simulink model "q_test_q2_usb"  (R2014b)
settings: Solver=FixedStepDiscrete  StartTime=0.0  StopTime=inf  FixedStep=0.002  RelTol=1e-3
PostLoadFcn:
  | qc_set_target_type(getConfigSet(bdroot, 'QUARC Default Target Configuration'));
undefined symbols (not defined in the file or in its folder): HIL, K_ENC, qc_get_step_size
libraries: quarc_library x12
settings Model: SimulationMode=external  ExtModeTrigDuration=5000  Creator=user  LastModifiedBy=amolki
settings SolverCC: PositivePriorityOrder=on
settings DataIOCC: SignalLoggingSaveFormat=ModelDataLogs
settings OptimizationCC: InitFltsAndDblsToZero=on
settings DebuggingCC: SaveWithParameterizedLinksMsg=none  UnderspecifiedInitializationDetection=Classic  MergeDetectMultiDrivingBlocksExec=none  MultiTaskDSMMsg=warning  MultiTaskCondExecSysMsg=none  FcnCallInpInsideContextMsg=UseLocalSettings  FrameProcessingCompatibilityMsg=error  StateNameClashWarn=warning
settings RTWCC: SystemTargetFile=quarc_win64.tlc  TemplateMakefile=quarc_default_tmf  Description=QUARC Win64 Target  ProcessScript=quarc_win64_make_rtw_hook
settings STFCustomTargetCC: TargetPreCompLibLocation=C:\PROGRA~3\QUARC\lib\2014b\win64\release  CodeReplacementLibrary=ANSI_C  ConcurrentExecutionCompliant=on  GeneratePreprocessorConditionals=Disable all  CombineOutputUpdateFcns=on  GRTInterface=off  SystemTargetFile=quarc_win64.tlc
settings GRTTargetCC: TargetPreCompLibLocation=C:\PROGRA~3\QUARC\lib\2014b\win64\release  CodeReplacementLibrary=ANSI_C  ParMdlRefBuildCompliant=off  CompOptLevelCompliant=off  MatFileLogging=off  CPPClassGenCompliant=off  ExtMode=on  ExtModeMexFile=quarc_comm

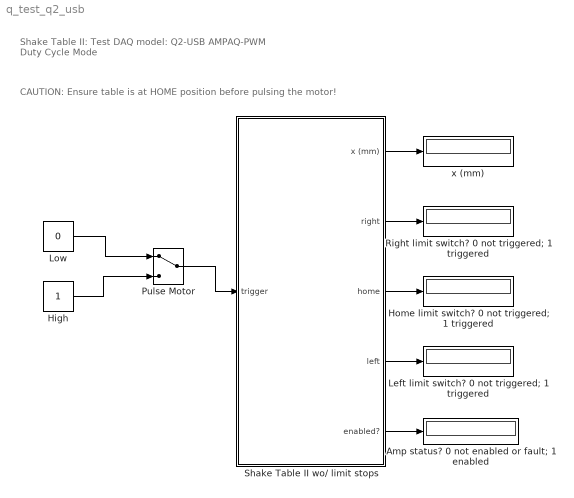
== system q_test_q2_usb ==
  note: Shake Table II: Test
      | DAQ model: Q2-USB
      | AMPAQ-PWM Duty Cycle Mode
  note: CAUTION: Ensure table is at HOME position before pulsing the motor!
  Amp status? 0 not enabled or fault; 1 enabled : Display
  High : Constant
  Home limit switch? 0 not triggered; 1 triggered : Display
  Left limit switch? 0 not triggered; 1 triggered : Display
  Low : Constant  Value=0
  Pulse Motor : ManualSwitch
  Right limit switch? 0 not triggered; 1 triggered : Display
  Shake Table II wo/ limit stops : Subsystem
  x (mm) : Display
  wires:
  Shake Table II wo/ limit stops/1(x (mm)) -> x (mm)/1
  Low/1 -> Pulse Motor/1
  High/1 -> Pulse Motor/2
  Shake Table II wo/ limit stops/2(right) -> Right limit switch? 0 not triggered; 1 triggered/1
  Shake Table II wo/ limit stops/4(left) -> Left limit switch? 0 not triggered; 1 triggered/1
  Shake Table II wo/ limit stops/3(home) -> Home limit switch? 0 not triggered; 1 triggered/1
  Shake Table II wo/ limit stops/5(enabled?) -> Amp status? 0 not enabled or fault; 1 enabled/1
  Pulse Motor/1 -> Shake Table II wo/ limit stops/1(trigger)

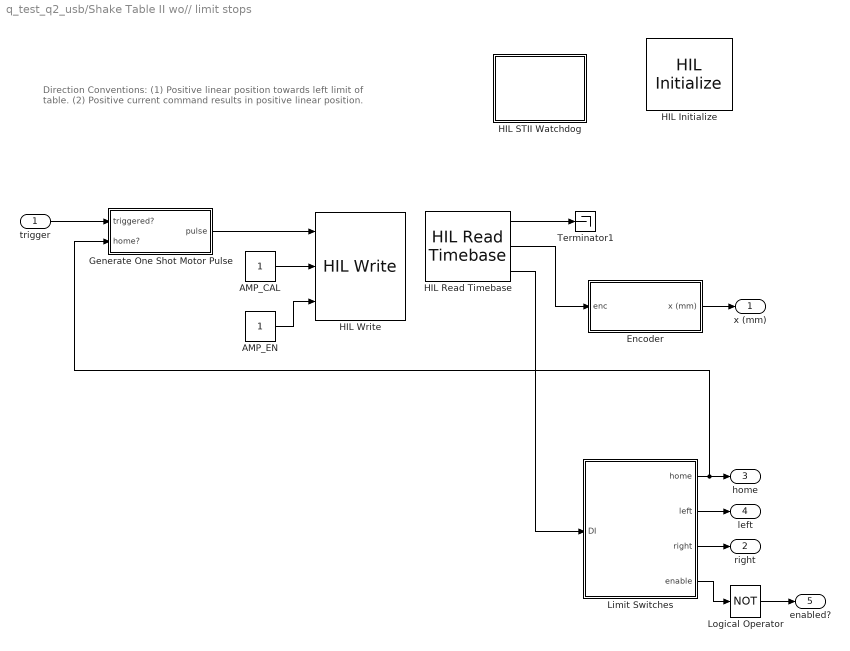
== system q_test_q2_usb/Shake Table II wo// limit stops ==
  note: Direction Conventions:
      | (1) Positive linear position towards left limit of table.
      | (2) Positive current command results in positive linear position.
  trigger : Inport
  AMP_CAL : Constant
  AMP_EN : Constant
  Encoder : Subsystem
  Generate One Shot Motor Pulse : Subsystem
  HIL Initialize : quarc_library/Data Acquisition/Generic/Configuration/HIL Initialize  object_name=HIL-1  board_type=q2_usb  board_number=0  board_options=d0=digital;d1=digital;led=auto;update_rate=fast;decimation=1  exclusive=off  active=on  hardware_clocks=[0]  clock_modes=[]  initial_clock_frequencies=[]  set_clock_params_at_start=off  set_clock_params_at_switch_in=off  set_clock_frequencies_at_start=off  set_clock_frequencies_at_switch_in=off  analog_input_channels=[0:1]  analog_input_maximums=10  analog_input_minimums=-10  set_analog_input_params_at_start=on  set_analog_input_params_at_switch_in=off  analog_output_channels=[0:1]  analog_output_maximums=10  analog_output_minimums=-10  initial_analog_outputs=[0]  final_analog_outputs=[0]  watchdog_analog_outputs=0  set_analog_output_params_at_start=on  set_analog_output_params_at_switch_in=off  set_analog_outputs_at_start=on  set_analog_outputs_at_switch_in=off  set_analog_outputs_at_terminate=on  set_analog_outputs_at_switch_out=off  set_analog_outputs_on_watchdog=off  digital_input_channels=[0:4]  digital_output_channels=[5:6]  digital_output_configuration=[]  initial_digital_outputs=[1]  final_digital_outputs=[1]  watchdog_digital_outputs=[1]  set_digital_output_params_at_start=off  set_digital_output_params_at_switch_in=off  set_digital_outputs_at_start=on  set_digital_outputs_at_switch_in=off  set_digital_outputs_at_terminate=on  set_digital_outputs_at_switch_out=off  set_digital_outputs_on_watchdog=off  encoder_channels=[0:1]  quadrature=[4]  encoder_filter_frequency=[]  initial_encoder_counts=[0]  set_encoder_params_at_start=on  set_encoder_params_at_switch_in=off  set_encoder_counts_at_start=on  set_encoder_counts_at_switch_in=off  pwm_channels=[]  pwm_modes=[0]  pwm_frequency=1/0.020  pwm_configuration=[]  pwm_alignment=[]  pwm_polarity=[]  pwm_leading_deadband=[]  pwm_trailing_deadband=[]  initial_pwm_outputs=[0]  final_pwm_outputs=[0]  watchdog_pwm_outputs=[0]  set_pwm_params_at_start=on  set_pwm_params_at_switch_in=off  set_pwm_outputs_at_start=on  set_pwm_outputs_at_switch_in=off  set_pwm_outputs_at_terminate=on  set_pwm_outputs_at_switch_out=off  set_pwm_outputs_on_watchdog=off  other_output_channels=[]  initial_other_outputs=[]  final_other_outputs=[]  watchdog_other_outputs=[]  set_other_outputs_at_start=off  set_other_outputs_at_switch_in=off  set_other_outputs_at_terminate=off  set_other_outputs_at_switch_out=off  set_other_outputs_on_watchdog=off
  HIL Read Timebase : quarc_library/Data Acquisition/Generic/Timebases/HIL Read Timebase  object_name=HIL-1  clock=0  analog_channels=[0:1]  encoder_channels=[0]  digital_channels=[0:4]  other_channels=[]  samples_in_buffer=max(ceil(1/qc_get_step_size), 1)  active=on  vector_output=on  data_type_mode=Inherit via back propagation  encoder_data_type=double  digital_data_type=boolean
  HIL STII Watchdog : Subsystem
  HIL Write : quarc_library/Data Acquisition/Generic/Immediate I//O/HIL Write  object_name=HIL-1  analog_channels=[0]  pwm_channels=[]  digital_channels=[5:6]  other_channels=[]  sample_time=-1  active=off  vector_input=off
  Limit Switches : Subsystem
  Logical Operator : Logic  Operator=NOT  AllPortsSameDT=off  OutDataTypeStr=boolean
  Terminator1 : Terminator
  x (mm) : Outport  InitialOutput=0
  right : Outport  Port=2  InitialOutput=0
  home : Outport  Port=3  InitialOutput=0
  left : Outport  Port=4  InitialOutput=0
  enabled? : Outport  Port=5
  wires:
  HIL Read Timebase/2 -> Encoder/1(enc)
  HIL Read Timebase/3 -> Limit Switches/1(DI)
  Encoder/1(x (mm)) -> x (mm)/1
  Limit Switches/1(home) -> Generate One Shot Motor Pulse/2(home?), home/1
  Limit Switches/2(left) -> left/1
  AMP_EN/1 -> HIL Write/3
  AMP_CAL/1 -> HIL Write/2
  Limit Switches/3(right) -> right/1
  HIL Read Timebase/1 -> Terminator1/1
  Logical Operator/1 -> enabled?/1
  trigger/1 -> Generate One Shot Motor Pulse/1(triggered?)
  Generate One Shot Motor Pulse/1(pulse) -> HIL Write/1
  Limit Switches/4(enable) -> Logical Operator/1

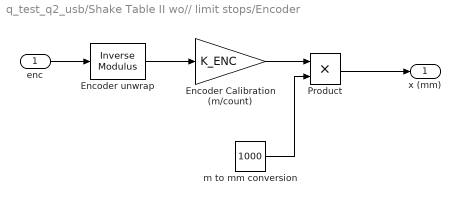
== system q_test_q2_usb/Shake Table II wo// limit stops/Encoder ==
  enc : Inport
  Encoder Calibration (m/count) : Gain  Gain=K_ENC  SaturateOnIntegerOverflow=on  OutDataTypeStr=Inherit: Same as input  ParamDataTypeStr=Inherit: Same as input
  Encoder unwrap : quarc_library/Discontinuities/Inverse Modulus  modulus=2^16  output_derivative=off  output_revolutions=off  max_x=Inf  min_x=-Inf
  Product : Product
  m to mm conversion : Constant  Value=1000
  x (mm) : Outport  InitialOutput=0
  wires:
  Product/1 -> x (mm)/1
  m to mm conversion/1 -> Product/2
  enc/1 -> Encoder unwrap/1
  Encoder Calibration (m/count)/1 -> Product/1
  Encoder unwrap/1 -> Encoder Calibration (m/count)/1

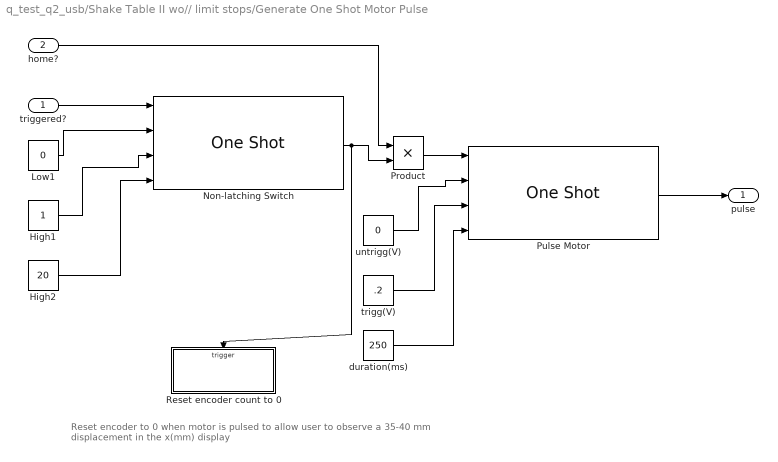
== system q_test_q2_usb/Shake Table II wo// limit stops/Generate One Shot Motor Pulse ==
  note: Reset encoder to 0 when motor is pulsed to
      | allow user to observe a 35-40 mm displacement in the x(mm) display
  triggered? : Inport
  home? : Inport  Port=2
  High1 : Constant
  High2 : Constant  Value=20
  Low1 : Constant  Value=0
  Non-latching Switch : quarc_library/Discontinuities/One Shot  trigger_type=Either edge  redun_pulse=Ignore extraneous pulse  width_source=External input port  pulse_width=1
  Product : Product
  Pulse Motor : quarc_library/Discontinuities/One Shot  trigger_type=Either edge  redun_pulse=Ignore extraneous pulse  width_source=External input port  pulse_width=1
  Reset encoder count to 0 : Subsystem  TreatAsAtomicUnit=on
  duration(ms) : Constant  Value=250
  trigg(V) : Constant  Value=.2
  untrigg(V) : Constant  Value=0
  pulse : Outport
  wires:
  triggered?/1 -> Non-latching Switch/1
  High1/1 -> Non-latching Switch/3
  Low1/1 -> Non-latching Switch/2
  High2/1 -> Non-latching Switch/4
  untrigg(V)/1 -> Pulse Motor/2
  trigg(V)/1 -> Pulse Motor/3
  duration(ms)/1 -> Pulse Motor/4
  Pulse Motor/1 -> pulse/1
  Product/1 -> Pulse Motor/1
  Non-latching Switch/1 -> Product/2, Reset encoder count to 0/Trigger
  home?/1 -> Product/1

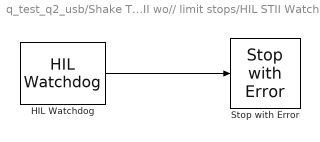
== system q_test_q2_usb/Shake Table II wo// limit stops/HIL STII Watchdog ==
  HIL Watchdog : quarc_library/Data Acquisition/Generic/Watchdog/HIL Watchdog  object_name=HIL-1  timeout=5*qc_get_step_size  sample_time=qc_get_step_size  active=off
      settings: AttributesFormatString=(%<object_name>)
  Stop with Error : quarc_library/Sinks/Error Handling/Stop with Error  message_type=Fixed error message  message=Stopped by Watchdog - controller began running too slow.
      settings: AttributesFormatString="\"%<message>\""
  wires:
  HIL Watchdog/1 -> Stop with Error/1

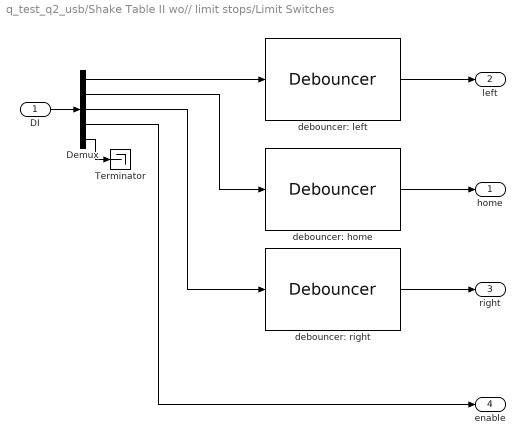
== system q_test_q2_usb/Shake Table II wo// limit stops/Limit Switches ==
  DI : Inport
  Demux : Demux  Outputs=5
  Terminator : Terminator
  debouncer: home : quarc_library/Discontinuities/Debouncer  init_state=Off  param_src=Specify via dialog  threshold=dbnc_threshold  rise_time=dbnc_rise_time  fall_time=0
  debouncer: left : quarc_library/Discontinuities/Debouncer  init_state=Off  param_src=Specify via dialog  threshold=dbnc_threshold  rise_time=dbnc_rise_time  fall_time=0
  debouncer: right : quarc_library/Discontinuities/Debouncer  init_state=Off  param_src=Specify via dialog  threshold=dbnc_threshold  rise_time=dbnc_rise_time  fall_time=0
  home : Outport
  left : Outport  Port=2
  right : Outport  Port=3
  enable : Outport  Port=4
  wires:
  debouncer: right/1 -> right/1
  Demux/3 -> debouncer: right/1
  DI/1 -> Demux/1
  Demux/1 -> debouncer: left/1
  debouncer: left/1 -> left/1
  Demux/2 -> debouncer: home/1
  debouncer: home/1 -> home/1
  Demux/4 -> enable/1
  Demux/5 -> Terminator/1

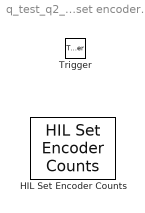
== system q_test_q2_usb/Shake Table II wo// limit stops/Generate One Shot Motor Pulse/Reset encoder count to 0 ==
  Trigger : TriggerPort
  HIL Set Encoder Counts : quarc_library/Data Acquisition/Generic/Configuration/HIL Set Encoder Counts  object_name=HIL-1  channels=0  source=internal  counts=0  sample_time=-1  active=on  vector_input=off
      settings: AttributesFormatString=(%<object_name>)
